simulink model "model3_first"  (R2022a)
settings: Solver=ode3  StartTime=0.0  StopTime=4  FixedStep=2e-6  MaxStep=2e-05  RelTol=1e-3
values from neighbouring files (symbols this model uses):
  c3_ = c3/(j23*j45*j67)^2    [EDriveLab1.m]
  c4_ = c4/(j23*j45*j67*j89)^2    [EDriveLab1.m]
  J10_2_ = m/2*(v/wd)^2    (= 1.61947385187e-05)    [EDriveLab1.m]
  J17_ = Jd + J2 + (J3+J4)/j23 + (J5+J6)/(j23*j45)+J7/(j23*j45*j67)    (= 0.594820647321)    [EDriveLab1.m]
  J810_ = J8/(j23*j45*j67) + J9/(j23*j45*j67*j89)+m/2*(v/wd)^2    (= 0.0578717345112)    [EDriveLab1.m]
  Md = m/2*10*v*(1+1/nc)/(wd*nr*nz*nz*nz*nv)    (= 6.52342119912)    [EDriveLab1.m]
undefined symbols (not defined in the file or in its folder): M_51new, M_52new
libraries: fl_lib x19, nesl_utility x9
settings Model: Creator=Elena  LastModifiedBy=Family
settings SolverCC: ZeroCrossAlgorithm=Adaptive  AlgebraicLoopSolver=TrustRegion
settings DataIOCC: ReturnWorkspaceOutputs=off
settings DebuggingCC: IgnoredZcDiagnostic=none  UnconnectedInputMsg=warning  UnconnectedOutputMsg=warning  UnconnectedLineMsg=warning  SFMachineParentedDataDiag=warning  ArithmeticOperatorsInVariantConditions=warning
settings SFSimCC: SimUseLocalCustomCode=off  CustomCodeUndefinedFunction=UseInterfaceOnly
settings RTWCC: RTWUseLocalCustomCode=off
settings CodeAppCC: StateflowObjectComments=on

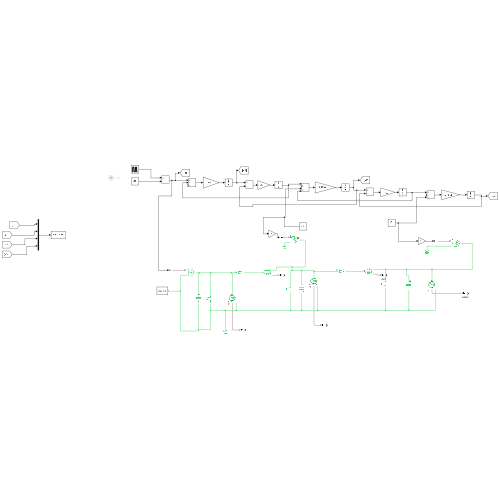
[thumbnail: Simulink's stored preview of the top-level diagram]
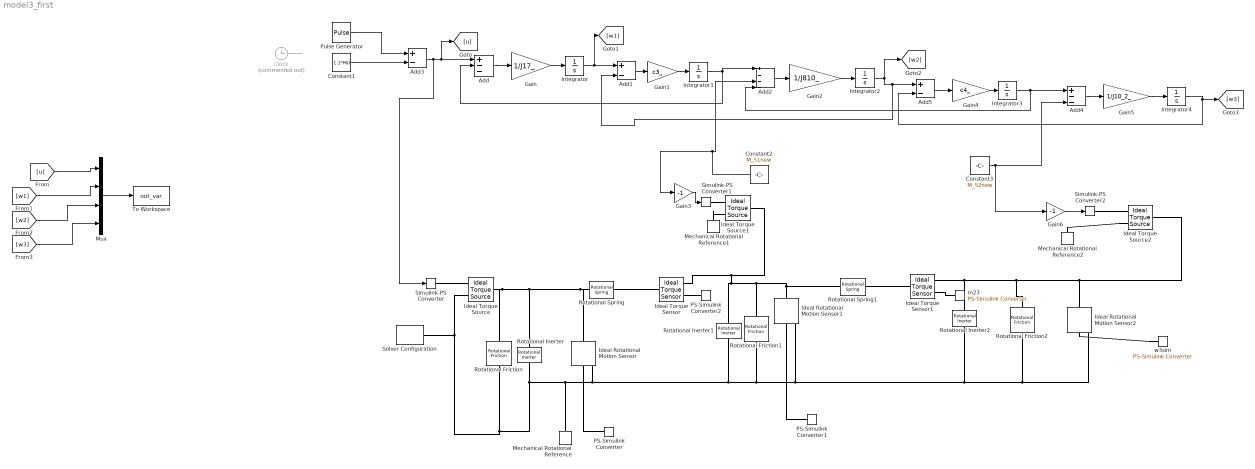
== system model3_first ==
  Add : Sum  Inputs=+--
  Add1 : Sum  Inputs=+-
  Add2 : Sum  Inputs=+---
  Add3 : Sum  Inputs=+-
  Add4 : Sum  Inputs=+--
  Add5 : Sum  Inputs=+-
  Clock : Clock  Commented=on
  Constant1 : Constant  Value=1.1*Md
  Constant2 : Constant  Value=M_51new
  Constant3 : Constant  Value=M_52new
  Gain : Gain  Gain=1/J17_
  Gain1 : Gain  Gain=c3_
  Gain2 : Gain  Gain=1/J810_
  Gain3 : Gain  Gain=-1
  Gain4 : Gain  Gain=c4_
  Gain5 : Gain  Gain=1/J10_2_
  Gain6 : Gain  Gain=-1
  Ideal Rotational Motion Sensor : fl_lib/Mechanical/Mechanical Sensors/Ideal Rotational Motion Sensor  wrap_angle=simscape.enum.onoff.off  offset=0 rad
      settings: SourceProductBaseCode=PW,SS,VE
  Ideal Rotational Motion Sensor1 : fl_lib/Mechanical/Mechanical Sensors/Ideal Rotational Motion Sensor  wrap_angle=simscape.enum.onoff.off  offset=0 rad
      settings: SourceProductBaseCode=PW,SS,VE
  Ideal Rotational Motion Sensor2 : fl_lib/Mechanical/Mechanical Sensors/Ideal Rotational Motion Sensor  wrap_angle=simscape.enum.onoff.off  offset=0 rad
      settings: SourceProductBaseCode=PW,SS,VE
  Ideal Torque Sensor : fl_lib/Mechanical/Mechanical Sensors/Ideal Torque Sensor
      settings: SourceProductBaseCode=PW,SS,VE
  Ideal Torque Sensor1 : fl_lib/Mechanical/Mechanical Sensors/Ideal Torque Sensor
      settings: SourceProductBaseCode=PW,SS,VE
  Ideal Torque Source : fl_lib/Mechanical/Mechanical Sources/Ideal Torque Source
      settings: SourceProductBaseCode=PW,SS,VE
  Ideal Torque Source1 : fl_lib/Mechanical/Mechanical Sources/Ideal Torque Source
      settings: SourceProductBaseCode=PW,SS,VE
  Ideal Torque Source2 : fl_lib/Mechanical/Mechanical Sources/Ideal Torque Source
      settings: SourceProductBaseCode=PW,SS,VE
  Integrator{,1..4} (5 alike) : Integrator
  Mechanical Rotational Reference : fl_lib/Mechanical/Rotational Elements/Mechanical Rotational Reference
      settings: SourceProductBaseCode=PW,SS,VE
  Mechanical Rotational Reference1 : fl_lib/Mechanical/Rotational Elements/Mechanical Rotational Reference
      settings: SourceProductBaseCode=PW,SS,VE
  Mechanical Rotational Reference2 : fl_lib/Mechanical/Rotational Elements/Mechanical Rotational Reference
      settings: SourceProductBaseCode=PW,SS,VE
  Mux : Mux
  PS-Simulink Converter : nesl_utility/PS-Simulink Converter  PhysicalDomain=network_engine_domain  SubClassName=ps_output  LeftPortType=input  RightPortType=output  PseudoPeriodic=off  Frequencies=[]  VectorFormat=1-D array  Unit=rad/s  AffineConversion=off
      settings: SourceProductBaseCode=SS,PW,VE
  PS-Simulink Converter1 : nesl_utility/PS-Simulink Converter  PhysicalDomain=network_engine_domain  SubClassName=ps_output  LeftPortType=input  RightPortType=output  PseudoPeriodic=off  Frequencies=[]  VectorFormat=1-D array  Unit=rad/s  AffineConversion=off
      settings: SourceProductBaseCode=SS,PW,VE
  PS-Simulink Converter2 : nesl_utility/PS-Simulink Converter  PhysicalDomain=network_engine_domain  SubClassName=ps_output  LeftPortType=input  RightPortType=output  PseudoPeriodic=off  Frequencies=[]  VectorFormat=1-D array  Unit=N*m  AffineConversion=off
      settings: SourceProductBaseCode=SS,PW,VE
  Pulse Generator : DiscretePulseGenerator  PulseType=Time based  Amplitude=2.2*Md  Period=1  PulseWidth=50
  Rotational Friction : fl_lib/Mechanical/Rotational Elements/Rotational Friction  brkwy_trq=Mf17_mass3 N*m  brkwy_vel=1e-06 rad/s  Col_trq=Mf17_mass3 N*m  visc_coef=0 N*m/(rad/s)  w_specify=off  w_priority=None  w=0 rad/s  w_nominal_specify=off  w_nominal_unit=rad/s  w_nominal_value=1  t_specify=off  t_priority=None  t=0 N*m  t_nominal_specify=off  t_nominal_unit=N*m  t_nominal_value=1
      settings: SourceProductBaseCode=PW,SS,VE
  Rotational Friction1 : fl_lib/Mechanical/Rotational Elements/Rotational Friction  brkwy_trq=Mf810_mass3 N*m  brkwy_vel=1e-06 rad/s  Col_trq=Mf810_mass3 N*m  visc_coef=0 N*m/(rad/s)  w_specify=off  w_priority=None  w=0 rad/s  w_nominal_specify=off  w_nominal_unit=rad/s  w_nominal_value=1  t_specify=off  t_priority=None  t=0 N*m  t_nominal_specify=off  t_nominal_unit=N*m  t_nominal_value=1
      settings: SourceProductBaseCode=PW,SS,VE
  Rotational Friction2 : fl_lib/Mechanical/Rotational Elements/Rotational Friction  brkwy_trq=Mf10_mass3 N*m  brkwy_vel=1e-06 rad/s  Col_trq=Mf10_mass3 N*m  visc_coef=0 N*m/(rad/s)  w_specify=off  w_priority=None  w=0 rad/s  w_nominal_specify=off  w_nominal_unit=rad/s  w_nominal_value=1  t_specify=off  t_priority=None  t=0 N*m  t_nominal_specify=off  t_nominal_unit=N*m  t_nominal_value=1
      settings: SourceProductBaseCode=PW,SS,VE
  Rotational Inerter : fl_lib/Mechanical/Rotational Elements/Rotational Inerter  B=J17_ kg*m^2  w_specify=off  w_priority=High  w=0 rad/s  w_nominal_specify=off  w_nominal_unit=rad/s  w_nominal_value=1  t_specify=off  t_priority=None  t=0 N*m  t_nominal_specify=off  t_nominal_unit=N*m  t_nominal_value=1
      settings: SourceProductBaseCode=PW,SS,VE  InternalSimscapePortConfiguration="{\"Bottom\":[],\"Left\":[{\"id\":\"R\",\"label\":\"R\",\"type\":\"foundation.mechanical.rotational.rotational\"}],\"Right\":[{\"id\":\"C\",\"label\":\"C\",\"type\":\"foundation.mechanical.rotational.rotational\"}],\"Top\":[]}"
  Rotational Inerter1 : fl_lib/Mechanical/Rotational Elements/Rotational Inerter  B=J810_ kg*m^2  w_specify=off  w_priority=High  w=0 rad/s  w_nominal_specify=off  w_nominal_unit=rad/s  w_nominal_value=1  t_specify=off  t_priority=None  t=0 N*m  t_nominal_specify=off  t_nominal_unit=N*m  t_nominal_value=1
      settings: SourceProductBaseCode=PW,SS,VE  InternalSimscapePortConfiguration="{\"Bottom\":[],\"Left\":[{\"id\":\"R\",\"label\":\"R\",\"type\":\"foundation.mechanical.rotational.rotational\"}],\"Right\":[{\"id\":\"C\",\"label\":\"C\",\"type\":\"foundation.mechanical.rotational.rotational\"}],\"Top\":[]}"
  Rotational Inerter2 : fl_lib/Mechanical/Rotational Elements/Rotational Inerter  B=J10_2_ kg*m^2  w_specify=off  w_priority=High  w=0 rad/s  w_nominal_specify=off  w_nominal_unit=rad/s  w_nominal_value=1  t_specify=off  t_priority=None  t=0 N*m  t_nominal_specify=off  t_nominal_unit=N*m  t_nominal_value=1
      settings: SourceProductBaseCode=PW,SS,VE  InternalSimscapePortConfiguration="{\"Bottom\":[],\"Left\":[{\"id\":\"R\",\"label\":\"R\",\"type\":\"foundation.mechanical.rotational.rotational\"}],\"Right\":[{\"id\":\"C\",\"label\":\"C\",\"type\":\"foundation.mechanical.rotational.rotational\"}],\"Top\":[]}"
  Rotational Spring : fl_lib/Mechanical/Rotational Elements/Rotational Spring  spr_rate=c3_ N*m/rad  w_specify=off  w_priority=None  w=0 rad/s  w_nominal_specify=off  w_nominal_unit=rad/s  w_nominal_value=1  t_specify=off  t_priority=None  t=0 N*m  t_nominal_specify=off  t_nominal_unit=N*m  t_nominal_value=1  phi_specify=off  phi_priority=High  phi=0 rad  phi_nominal_specify=off  phi_nominal_unit=rad  phi_nominal_value=1
      settings: SourceProductBaseCode=PW,SS,VE
  Rotational Spring1 : fl_lib/Mechanical/Rotational Elements/Rotational Spring  spr_rate=c4_ N*m/rad  w_specify=off  w_priority=None  w=0 rad/s  w_nominal_specify=off  w_nominal_unit=rad/s  w_nominal_value=1  t_specify=off  t_priority=None  t=0 N*m  t_nominal_specify=off  t_nominal_unit=N*m  t_nominal_value=1  phi_specify=off  phi_priority=High  phi=0 rad  phi_nominal_specify=off  phi_nominal_unit=rad  phi_nominal_value=1
      settings: SourceProductBaseCode=PW,SS,VE
  Simulink-PS Converter : nesl_utility/Simulink-PS Converter  PhysicalDomain=network_engine_domain  SubClassName=ps_input  LeftPortType=input  RightPortType=output  PseudoPeriodic=off  Frequencies=[]  NoiseDistribution=none  NoiseParameters=[]  Unit=1  AffineConversion=off  FilteringAndDerivatives=provide  SimscapeFilterOrder=1  InputFilterTimeConstant=2e-5  UdotUserProvided=0
      settings: SourceProductBaseCode=SS,PW,VE
  Simulink-PS Converter1 : nesl_utility/Simulink-PS Converter  PhysicalDomain=network_engine_domain  SubClassName=ps_input  LeftPortType=input  RightPortType=output  PseudoPeriodic=off  Frequencies=[]  NoiseDistribution=none  NoiseParameters=[]  Unit=1  AffineConversion=off  FilteringAndDerivatives=provide  SimscapeFilterOrder=1  InputFilterTimeConstant=0.001  UdotUserProvided=0
      settings: SourceProductBaseCode=SS,PW,VE
  Simulink-PS Converter2 : nesl_utility/Simulink-PS Converter  PhysicalDomain=network_engine_domain  SubClassName=ps_input  LeftPortType=input  RightPortType=output  PseudoPeriodic=off  Frequencies=[]  NoiseDistribution=none  NoiseParameters=[]  Unit=1  AffineConversion=off  FilteringAndDerivatives=provide  SimscapeFilterOrder=1  InputFilterTimeConstant=0.001  UdotUserProvided=0
      settings: SourceProductBaseCode=SS,PW,VE
  Solver Configuration : nesl_utility/Solver Configuration  PhysicalDomain=network_engine_domain  SubClassName=solver  LeftPortType=input  RightPortType=generic  Tones=[]  Harmonics=[]  SimulateNoise=off  Profile=off  UseLocalSampling=off  EnableSwitchedLinearOptims=on  FrequencyDomain=off  UseCCode=off  RelTol=0.001  AbsTol=1e-06  MinStep=1e-09  ToWorkspace=off  RevertToSquareIcSolve=off  NumHomotopyIterations=100  PhasorMode=off  PhasorModeNumHarmonics=1  IndexReductionMethod=DerivativeReplacement  DoDC=off  ResidualTolerance=1e-09  UseLocalSolver=on  LocalSolverChoice=NE_TRAPEZOIDAL_ADVANCER  LocalSolverSampleTime=1e-5  DoFixedCost=on  MaxNonlinIter=3  MaxModeIter=2  ComputeImpulses=off  ImpulseIterations=2  LinearAlgebra=Sparse  LinearAlgebraNumThread=0  EquationFormulation=NE_TIME_EF  DelaysMemoryBudget=1024  AutomaticFiltering=on  FilteringTimeConstant=0.001  PartitionStorageMethod=AS_NEEDED  PartitionMemoryBudget=1024  PartitionMethod=FAST
      settings: SourceProductBaseCode=SS,PW,VE
  To Workspace : ToWorkspace  VariableName=out_var  SaveFormat=Structure With Time  SampleTime=0.001
  m23 : nesl_utility/PS-Simulink Converter  PhysicalDomain=network_engine_domain  SubClassName=ps_output  LeftPortType=input  RightPortType=output  PseudoPeriodic=off  Frequencies=[]  VectorFormat=1-D array  Unit=N*m  AffineConversion=off
      settings: SourceProductBaseCode=SS,PW,VE
  w3sim : nesl_utility/PS-Simulink Converter  PhysicalDomain=network_engine_domain  SubClassName=ps_output  LeftPortType=input  RightPortType=output  PseudoPeriodic=off  Frequencies=[]  VectorFormat=1-D array  Unit=rad/s  AffineConversion=off
      settings: SourceProductBaseCode=SS,PW,VE
  wires:
  Gain/1 -> Integrator/1
  Gain1/1 -> Integrator1/1
  Gain2/1 -> Integrator2/1
  Add/1 -> Gain/1
  Pulse Generator/1 -> Add3/1
  Constant1/1 -> Add3/2
  Add3/1 -> Simulink-PS Converter/1, [u], Add/1
  Add1/1 -> Gain1/1
  Integrator1/1 -> Add/2, Add2/1
  Add2/1 -> Gain2/1
  Integrator2/1 -> Add5/1, Add1/2, [w2]
  Mux/1 -> To Workspace/1
  Integrator/1 -> [w1], Add1/1
  [u] -> Mux/1
  [w1] -> Mux/2
  [w2] -> Mux/3
  Clock/1 -> ?
  Constant2/1 -> Gain3/1, Add2/3
  Gain3/1 -> Simulink-PS Converter1/1
  Gain4/1 -> Integrator3/1
  Add5/1 -> Gain4/1
  Integrator3/1 -> Add2/4, Add4/1
  Add4/1 -> Gain5/1
  Gain5/1 -> Integrator4/1
  Integrator4/1 -> [w3], Add5/2
  Constant3/1 -> Add4/3, Gain6/1
  [w3] -> Mux/4
  Gain6/1 -> Simulink-PS Converter2/1
  connections:
  Simulink-PS Converter/RConn1 -- Ideal Torque Source/RConn1
  Ideal Torque Source/LConn1 -- Rotational Friction/LConn1 -- Ideal Rotational Motion Sensor/LConn1 -- Rotational Spring/LConn1 -- Rotational Inerter/LConn1
  Mechanical Rotational Reference/LConn1 -- Ideal Rotational Motion Sensor/RConn1 -- Ideal Rotational Motion Sensor1/RConn1 -- Rotational Friction2/RConn1 -- Ideal Rotational Motion Sensor2/RConn1 -- Rotational Inerter2/RConn1 -- Rotational Friction1/RConn1 -- Rotational Inerter1/RConn1 -- Rotational Friction/RConn1 -- Solver Configuration/RConn1 -- Ideal Torque Source/RConn2 -- Rotational Inerter/RConn1
  Ideal Torque Sensor/LConn1 -- Rotational Spring/RConn1
  Ideal Torque Sensor/RConn1 -- Ideal Torque Source1/LConn1 -- Rotational Spring1/LConn1 -- Ideal Rotational Motion Sensor1/LConn1 -- Rotational Friction1/LConn1 -- Rotational Inerter1/LConn1
  PS-Simulink Converter/LConn1 -- Ideal Rotational Motion Sensor/RConn2
  PS-Simulink Converter1/LConn1 -- Ideal Rotational Motion Sensor1/RConn2
  PS-Simulink Converter2/LConn1 -- Ideal Torque Sensor/RConn2
  Simulink-PS Converter1/RConn1 -- Ideal Torque Source1/RConn1
  Mechanical Rotational Reference1/LConn1 -- Ideal Torque Source1/RConn2
  Rotational Spring1/RConn1 -- Ideal Torque Sensor1/LConn1
  Ideal Torque Sensor1/RConn1 -- Ideal Torque Source2/LConn1 -- Ideal Rotational Motion Sensor2/LConn1 -- Rotational Friction2/LConn1 -- Rotational Inerter2/LConn1
  w3sim/LConn1 -- Ideal Rotational Motion Sensor2/RConn2
  m23/LConn1 -- Ideal Torque Sensor1/RConn2
  Simulink-PS Converter2/RConn1 -- Ideal Torque Source2/RConn1
  Ideal Torque Source2/RConn2 -- Mechanical Rotational Reference2/LConn1
